simulink model "autoArrange"  (R2022b)
settings: Solver=VariableStepAuto  StartTime=0.0  StopTime=100.0  RelTol=1e-3
settings Model: Creator=YJT  LastModifiedBy=YJT

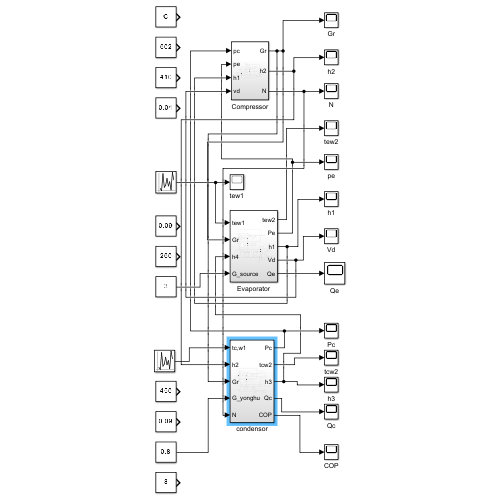
[thumbnail: Simulink's stored preview of the top-level diagram]
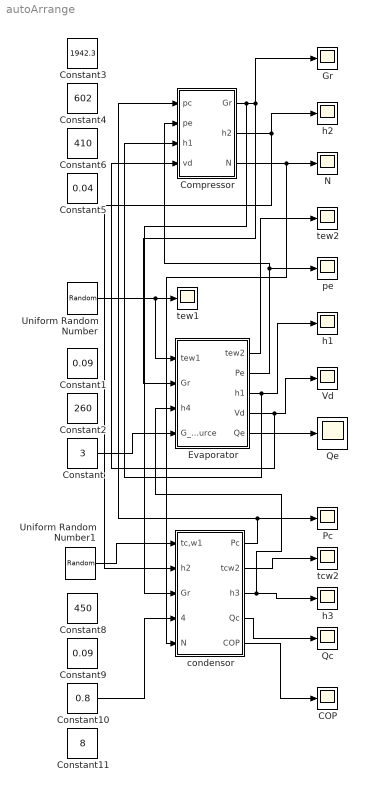
== system autoArrange ==
  COP : Scope
  Compressor : Subsystem
  Constant : Constant  Value=3
  Constant1 : Constant  Value=0.09
  Constant10 : Constant  Value=0.8
  Constant11 : Constant  Value=8
  Constant2 : Constant  Value=260
  Constant3 : Constant  Value=1942.3
  Constant4 : Constant  Value=602
  Constant5 : Constant  Value=0.04
  Constant6 : Constant  Value=410
  Constant8 : Constant  Value=450
  Constant9 : Constant  Value=0.09
  Evaporator : Subsystem
  Gr : Scope
  N : Scope
  Pc : Scope
  Qc : Scope
  Qe : Scope
  Uniform Random Number : UniformRandomNumber  Minimum=11  Maximum=12  SampleTime=0.1
  Uniform Random Number1 : UniformRandomNumber  Minimum=35  Maximum=38  SampleTime=0.1
  Vd : Scope
  condensor : Subsystem
  h1 : Scope
  h2 : Scope
  h3 : Scope
  pe : Scope
  tcw2 : Scope
  tew1 : Scope
  tew2 : Scope
  wires:
  Constant/1 -> Evaporator/4(G_source)
  Constant10/1 -> condensor/4(G_yonghu)
  condensor/5(COP) -> COP/1
  Uniform Random Number/1 -> Evaporator/1(tew1), tew1/1
  condensor/4(Qc) -> Qc/1
  Uniform Random Number1/1 -> condensor/1(tc,w1)
  condensor/2(tcw2) -> tcw2/1
  Compressor/1(Gr) -> condensor/3(Gr), Evaporator/2(Gr), Gr/1
  Compressor/2(h2) -> condensor/2(h2), h2/1
  Compressor/3(N) -> condensor/5(N), N/1
  Evaporator/2(Pe) -> Compressor/2(pe), pe/1
  Evaporator/1(tew2) -> tew2/1
  Evaporator/5(Qe) -> Qe/1
  Evaporator/4(Vd) -> Compressor/4(vd), Vd/1
  Evaporator/3(h1) -> Compressor/3(h1), h1/1
  condensor/1(Pc) -> Compressor/1(pc), Pc/1
  condensor/3(h3) -> Evaporator/3(h4), h3/1

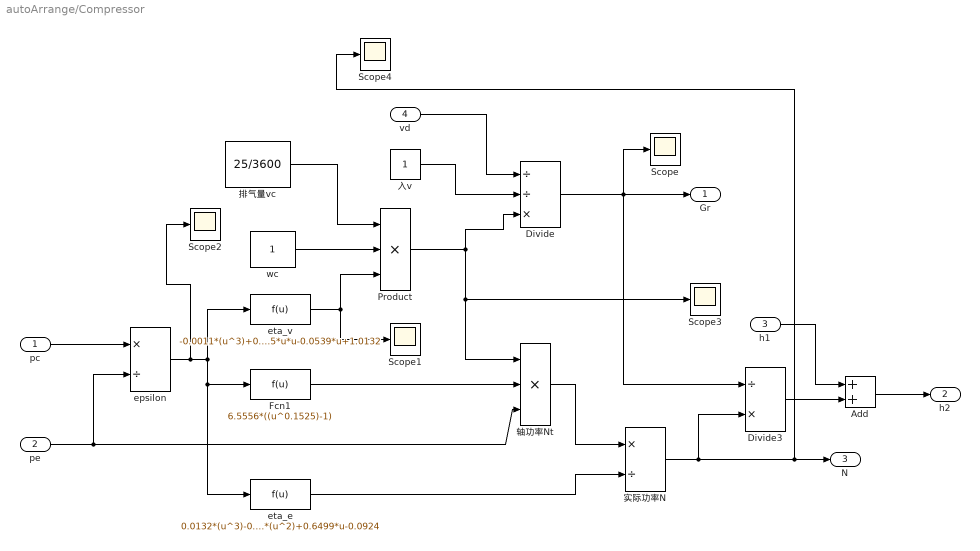
== system autoArrange/Compressor ==
  pc : Inport
  pe : Inport  Port=2
  h1 : Inport  Port=3
  vd : Inport  Port=4
  Add : Sum
  Divide : Product  Inputs=//*
  Divide3 : Product  Inputs=/*
  Fcn1 : Fcn  Expr=6.5556*((u^0.1525)-1)
  Product : Product  Inputs=3
  Scope{,1..4} (5 alike) : Scope
  epsilon : Product  Inputs=*/
  eta_e : Fcn  Expr=0.0132*(u^3)-0.1677*(u^2)+0.6499*u-0.0924
  eta_v : Fcn  Expr=-0.0011*(u^3)+0.0105*u*u-0.0539*u+1.0132
  wc : Constant
  入v : Constant
  实际功率N : Product  Inputs=*/
  排气量vc : Constant  Value=25/3600
  轴功率Nt : Product  Inputs=3
  Gr : Outport
  h2 : Outport  Port=2
  N : Outport  Port=3
  wires:
  排气量vc/1 -> Product/1
  Divide/1 -> Divide3/1, Scope/1, Gr/1
  Fcn1/1 -> 轴功率Nt/2
  轴功率Nt/1 -> 实际功率N/1
  epsilon/1 -> Scope2/1, eta_e/1, Fcn1/1, eta_v/1
  pc/1 -> epsilon/1
  eta_v/1 -> Product/3, Scope1/1
  Add/1 -> h2/1
  入v/1 -> Divide/2
  eta_e/1 -> 实际功率N/2
  wc/1 -> Product/2
  Product/1 -> Scope3/1, 轴功率Nt/1, Divide/3
  实际功率N/1 -> Scope4/1, N/1, Divide3/2
  Divide3/1 -> Add/2
  pe/1 -> epsilon/2, 轴功率Nt/3
  h1/1 -> Add/1
  vd/1 -> Divide/1

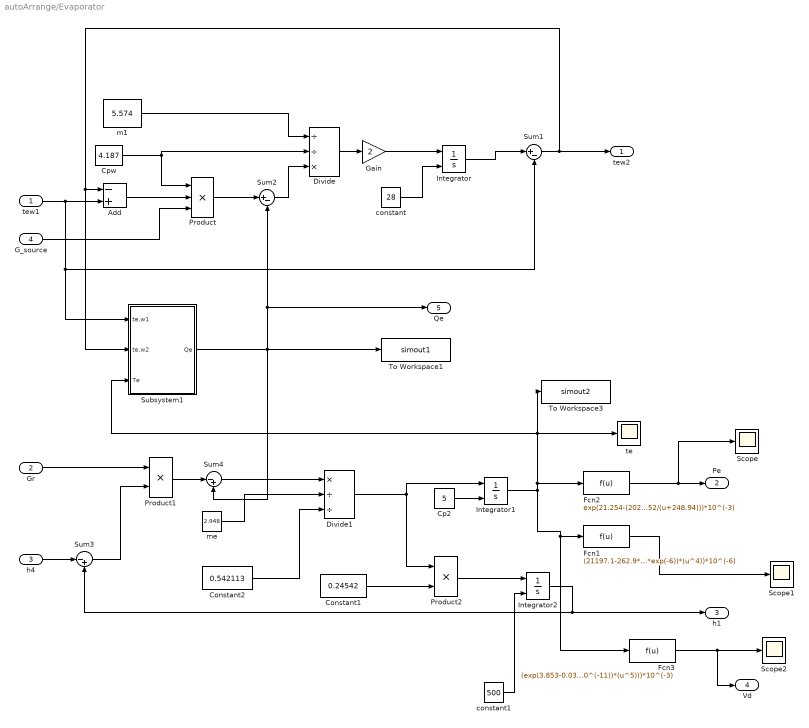
== system autoArrange/Evaporator ==
  tew1 : Inport
  Gr : Inport  Port=2
  h4 : Inport  Port=3
  G_source : Inport  Port=4
  Add : Sum  Inputs=-+
  Constant1 : Constant  Value=0.24542
  Constant2 : Constant  Value=0.542113
  Cp2 : Constant  Value=5
  Cpw : Constant  Value=4.187
  Divide : Product  Inputs=//*
  Divide1 : Product  Inputs=*//
  Fcn1 : Fcn  Expr=(21197.1-262.9*u+1.232*(u^2)-0.0026*(u^3)+(2.033*exp(-6))*(u^4))*10^(-6)
  Fcn2 : Fcn  Expr=exp(21.254-(2025.452/(u+248.94)))*10^(-3)
  Fcn3 : Fcn  Expr=(exp(3.853-0.031563*u+10.3312*(10^(-5))*(u^2)-6.2779*(10^(-7))*(u^3)+1.374867*(10^(-9))*(u^4)-2.07723*(10^(-11))*(u^5)))*10^(-3)
  Gain : Gain  Gain=2
  Integrator : Integrator  InitialConditionSource=external
  Integrator1 : Integrator  InitialConditionSource=external
  Integrator2 : Integrator  InitialConditionSource=external
  Product : Product  Inputs=3
  Product1 : Product
  Product2 : Product
  Scope : Scope
  Scope1 : Scope
  Scope2 : Scope
  Subsystem1 : Subsystem
  Sum1 : Sum  Inputs=|+-
  Sum2 : Sum  Inputs=|+-
  Sum3 : Sum  Inputs=|-+
  Sum4 : Sum  Inputs=|-+
  To Workspace1 : ToWorkspace  VariableName=simout1  SaveFormat=Timeseries  SampleTime=-1
  To Workspace3 : ToWorkspace  VariableName=simout2  SaveFormat=Timeseries  SampleTime=-1
  constant : Constant  Value=28
  constant1 : Constant  Value=500
  m1 : Constant  Value=5.574
  me : Constant  Value=2.948
  te : Scope
  tew2 : Outport
  Pe : Outport  Port=2
  h1 : Outport  Port=3
  Vd : Outport  Port=4
  Qe : Outport  Port=5
  wires:
  h4/1 -> Sum3/1
  Constant2/1 -> Divide1/3
  tew1/1 -> Add/2, Subsystem1/1(te,w1), Sum1/2
  Product1/1 -> Sum4/1
  Sum1/1 -> tew2/1, Subsystem1/2(te,w2), Add/1
  Product/1 -> Sum2/1
  Gr/1 -> Product1/1
  Fcn1/1 -> Scope1/1
  G_source/1 -> Product/3
  Cpw/1 -> Divide/2, Product/1
  Integrator2/1 -> h1/1, Sum3/2
  Divide1/1 -> Product2/1, Integrator1/1
  Sum3/1 -> Product1/2
  Sum4/1 -> Divide1/1
  Constant1/1 -> Product2/2
  m1/1 -> Divide/1
  Fcn2/1 -> Scope/1, Pe/1
  Add/1 -> Product/2
  Integrator1/1 -> te/1, Subsystem1/3(Te), To Workspace3/1, Fcn2/1, Fcn3/1, Fcn1/1
  Product2/1 -> Integrator2/1
  Sum2/1 -> Divide/3
  Divide/1 -> Gain/1
  Cp2/1 -> Integrator1/2
  Subsystem1/1(Qe) -> Qe/1, Sum2/2, Sum4/2, To Workspace1/1
  me/1 -> Divide1/2
  constant/1 -> Integrator/2
  Gain/1 -> Integrator/1
  Integrator/1 -> Sum1/1
  constant1/1 -> Integrator2/2
  Fcn3/1 -> Vd/1, Scope2/1

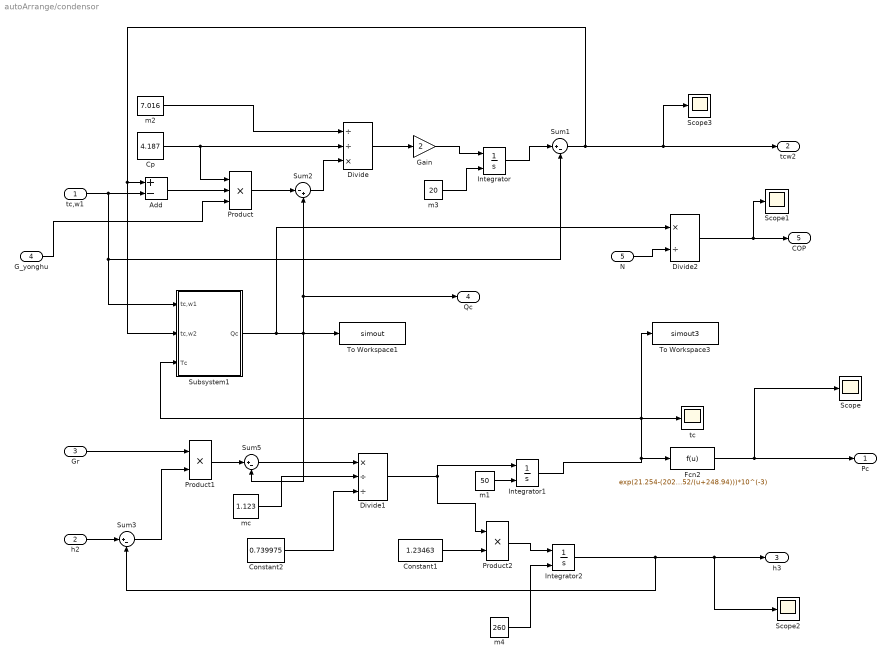
== system autoArrange/condensor ==
  tc,w1 : Inport
  h2 : Inport  Port=2
  Gr : Inport  Port=3
  G_yonghu : Inport  Port=4
  N : Inport  Port=5
  Add : Sum  Inputs=+-
  Constant1 : Constant  Value=1.23463
  Constant2 : Constant  Value=0.739975
  Cp : Constant  Value=4.187
  Divide : Product  Inputs=//*
  Divide1 : Product  Inputs=*//
  Divide2 : Product  Inputs=*/
  Fcn2 : Fcn  Expr=exp(21.254-(2025.452/(u+248.94)))*10^(-3)
  Gain : Gain  Gain=2
  Integrator : Integrator  InitialConditionSource=external
  Integrator1 : Integrator  InitialConditionSource=external
  Integrator2 : Integrator  InitialConditionSource=external
  Product : Product  Inputs=3
  Product1 : Product
  Product2 : Product
  Scope{,1..3} (4 alike) : Scope
  Subsystem1 : Subsystem
  Sum1 : Sum  Inputs=|+-
  Sum2 : Sum  Inputs=|-+
  Sum3 : Sum  Inputs=|+-
  Sum5 : Sum  Inputs=|+-
  To Workspace1 : ToWorkspace  VariableName=simout  SaveFormat=Timeseries  SampleTime=-1
  To Workspace3 : ToWorkspace  VariableName=simout3  SaveFormat=Timeseries  SampleTime=-1
  m1 : Constant  Value=50
  m2 : Constant  Value=7.016
  m3 : Constant  Value=20
  m4 : Constant  Value=260
  mc : Constant  Value=1.123
  tc : Scope
  Pc : Outport
  tcw2 : Outport  Port=2
  h3 : Outport  Port=3
  Qc : Outport  Port=4
  COP : Outport  Port=5
  wires:
  Product1/1 -> Sum5/1
  Sum3/1 -> Product1/2
  Sum1/1 -> Scope3/1, tcw2/1, Subsystem1/2(tc,w2), Add/1
  Gr/1 -> Product1/1
  Integrator2/1 -> Scope2/1, h3/1, Sum3/2
  Constant2/1 -> Divide1/3
  Gain/1 -> Integrator/1
  tc,w1/1 -> Add/2, Subsystem1/1(tc,w1), Sum1/2
  Fcn2/1 -> Scope/1, Pc/1
  Product2/1 -> Integrator2/1
  Integrator/1 -> Sum1/1
  m2/1 -> Divide/1
  Cp/1 -> Product/1, Divide/2
  Constant1/1 -> Product2/2
  G_yonghu/1 -> Product/3
  Divide1/1 -> Integrator1/1, Product2/1
  Divide/1 -> Gain/1
  h2/1 -> Sum3/1
  Product/1 -> Sum2/1
  Add/1 -> Product/2
  Sum5/1 -> Divide1/1
  Sum2/1 -> Divide/3
  mc/1 -> Divide1/2
  m1/1 -> Integrator1/2
  Integrator1/1 -> tc/1, To Workspace3/1, Subsystem1/3(Tc), Fcn2/1
  m3/1 -> Integrator/2
  m4/1 -> Integrator2/2
  Divide2/1 -> Scope1/1, COP/1
  Subsystem1/1(Qc) -> Divide2/1, Sum5/2, Qc/1, Sum2/2, To Workspace1/1
  N/1 -> Divide2/2

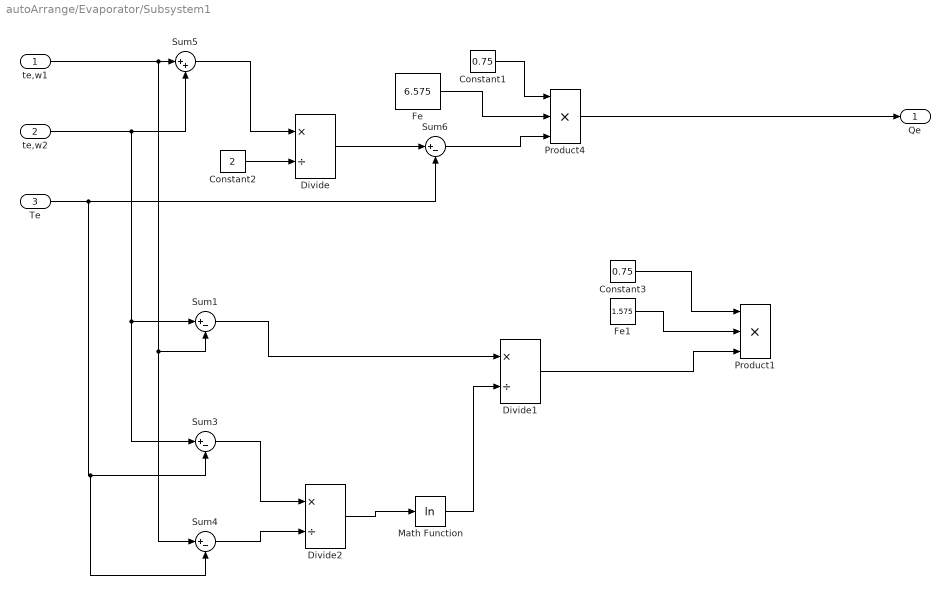
== system autoArrange/Evaporator/Subsystem1 ==
  te,w1 : Inport
  te,w2 : Inport  Port=2
  Te : Inport  Port=3
  Constant1 : Constant  Value=0.75
  Constant2 : Constant  Value=2
  Constant3 : Constant  Value=0.75
  Divide : Product  Inputs=*/
  Divide1 : Product  Inputs=*/
  Divide2 : Product  Inputs=*/
  Fe : Constant  Value=6.575
  Fe1 : Constant  Value=1.575
  Math Function : Math  Operator=log
  Product1 : Product  Inputs=3
  Product4 : Product  Inputs=3
  Sum{1,3..4,6} (4 alike) : Sum  Inputs=|+-
  Sum5 : Sum  Inputs=|++
  Qe : Outport
  wires:
  te,w2/1 -> Sum5/2, Sum1/1, Sum3/1
  Divide/1 -> Sum6/1
  Fe/1 -> Product4/2
  Sum6/1 -> Product4/3
  Sum5/1 -> Divide/1
  te,w1/1 -> Sum4/1, Sum1/2, Sum5/1
  Constant1/1 -> Product4/1
  Constant2/1 -> Divide/2
  Sum1/1 -> Divide1/1
  Constant3/1 -> Product1/1
  Fe1/1 -> Product1/2
  Divide1/1 -> Product1/3
  Te/1 -> Sum6/2, Sum4/2, Sum3/2
  Sum3/1 -> Divide2/1
  Sum4/1 -> Divide2/2
  Divide2/1 -> Math Function/1
  Math Function/1 -> Divide1/2
  Product4/1 -> Qe/1

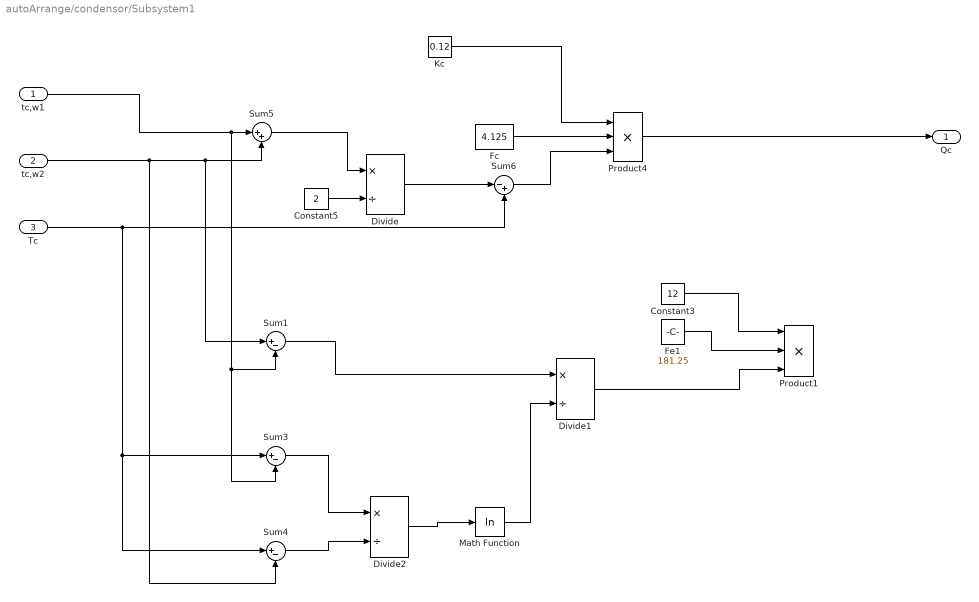
== system autoArrange/condensor/Subsystem1 ==
  tc,w1 : Inport
  tc,w2 : Inport  Port=2
  Tc : Inport  Port=3
  Constant3 : Constant  Value=12
  Constant5 : Constant  Value=2
  Divide : Product  Inputs=*/
  Divide1 : Product  Inputs=*/
  Divide2 : Product  Inputs=*/
  Fc : Constant  Value=4.125
  Fe1 : Constant  Value=181.25
  Kc : Constant  Value=0.12
  Math Function : Math  Operator=log
  Product1 : Product  Inputs=3
  Product4 : Product  Inputs=3
  Sum1 : Sum  Inputs=|+-
  Sum3 : Sum  Inputs=|+-
  Sum4 : Sum  Inputs=|+-
  Sum5 : Sum  Inputs=|++
  Sum6 : Sum  Inputs=|-+
  Qc : Outport
  wires:
  Divide/1 -> Sum6/1
  Fc/1 -> Product4/2
  Sum6/1 -> Product4/3
  Tc/1 -> Sum4/1, Sum3/1, Sum6/2
  Constant5/1 -> Divide/2
  Kc/1 -> Product4/1
  Sum5/1 -> Divide/1
  Sum3/1 -> Divide2/1
  Divide2/1 -> Math Function/1
  tc,w1/1 -> Sum3/2, Sum1/2, Sum5/1
  Sum1/1 -> Divide1/1
  Fe1/1 -> Product1/2
  Constant3/1 -> Product1/1
  Sum4/1 -> Divide2/2
  Divide1/1 -> Product1/3
  tc,w2/1 -> Sum4/2, Sum1/1, Sum5/2
  Math Function/1 -> Divide1/2
  Product4/1 -> Qc/1
